simulink model "mdaqdemo_ext"  (R2013a)
settings: Solver=FixedStepDiscrete  StartTime=0.0  StopTime=inf  RelTol=1e-3
PostLoadFcn:
  | set_param(gcs,'OnTargetWaitForStart','on');
settings Model: SimulationMode=external  ExtModeTrigDuration=100  Creator=peselnikmg  LastModifiedBy=peselnikmg
settings DataIOCC: SignalLoggingSaveFormat=ModelDataLogs
settings OptimizationCC: OptimizeModelRefInitCode=on  LifeSpan=1
settings HardwareCC: ProdBitPerLong=40  ProdLargestAtomicInteger=Integer  ProdIntDivRoundTo=Zero  ProdEndianess=LittleEndian  ProdHWDeviceType=Texas Instruments->C6000
settings RTWCC: SystemTargetFile=microdaq.tlc  TemplateMakefile=microdaq.tmf  PostCodeGenCommand=microdaq_postcodegen(buildInfo)  Description=MicroDAQ Real-Time Measurement System  GenerateReport=on  ProcessScript=microdaq_make_rtw_hook  IncludeHyperlinkInReport=on
settings CodeAppCC: IgnoreCustomStorageClasses=off
settings STFCustomTargetCC: CodeReplacementLibrary=TI C674x  CombineOutputUpdateFcns=on  ERTCustomFileBanners=on  SupportContinuousTime=off  SupportNonInlinedSFcns=off  MATLABClassNameForMDSCustomization=Simulink.SoftwareTarget.ERTCustomization  SystemTargetFile=microdaq.tlc
settings ERTTargetCC: CodeReplacementLibrary=TI C674x  GenerateSampleERTMain=off  ParMdlRefBuildCompliant=off  CompOptLevelCompliant=off  ConcurrentExecutionCompliant=off  ERTFirstTimeCompliant=off  ModelStepFunctionPrototypeControlCompliant=off  CPPClassGenCompliant=off  ExtMode=on  ExtModeMexFile=ext_mdaq_mlink  ExtModeMexArgs=1 getpref('microdaq','TargetIP')  ERTCustomFileTemplate=microdaq_main.tlc

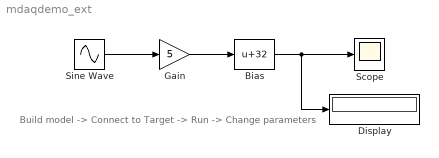
== system mdaqdemo_ext ==
  note: Build model -> Connect to Target ->
      | Run -> Change parameters
  Bias : Bias  Bias=32
  Display : Display
  Gain : Gain  Gain=5
  Scope : Scope
      settings: TimeRange=10  YMin=27  YMax=37  MaxDataPoints=10
  Sine Wave : Sin  SampleTime=0.1
  wires:
  Sine Wave/1 -> Gain/1
  Bias/1 -> Display/1, Scope/1
  Gain/1 -> Bias/1
